simulink model "sim_yawrate"  (R2022b)
settings: Solver=VariableStepAuto  StartTime=0.0  StopTime=10.0  RelTol=1e-3
libraries: cstblocks x1
settings Model: Creator=studenti  LastModifiedBy=tonegas
settings SolverCC: AlgebraicLoopSolver=TrustRegion
settings DebuggingCC: UnconnectedInputMsg=warning  UnconnectedOutputMsg=warning  UnconnectedLineMsg=warning  SFMachineParentedDataDiag=warning
settings ModelReferenceCC: EnableRefExpFcnMdlSchedulingChecks=on

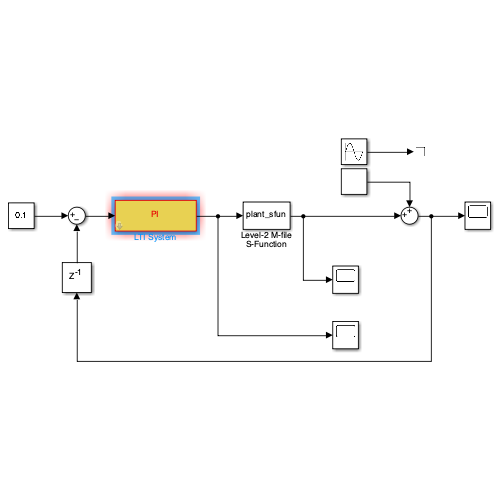
[thumbnail: Simulink's stored preview of the top-level diagram]
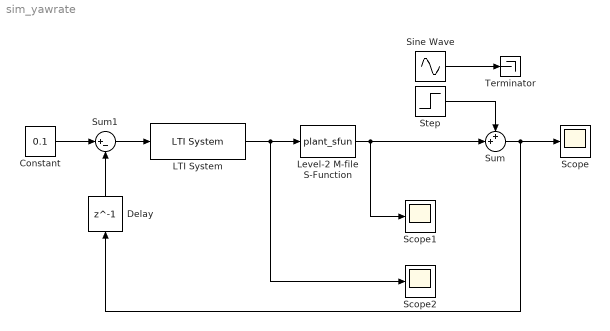
== system sim_yawrate ==
  Constant : Constant  Value=0.1
  Delay : Delay  DelayLength=1  InitialCondition=0
  LTI System : cstblocks/LTI System  sys=PI  IC=[]
  Level-2 M-file S-Function : M-S-Function  FunctionName=plant_sfun
  Scope : Scope
  Scope1 : Scope
  Scope2 : Scope
  Sine Wave : Sin  Frequency=0.5  SampleTime=0
  Step : Step  After=0.05  SampleTime=0
  Sum : Sum  Inputs=++|
  Sum1 : Sum  Inputs=|+-
  Terminator : Terminator
  wires:
  LTI System/1 -> Level-2 M-file S-Function/1, Scope2/1
  Constant/1 -> Sum1/1
  Level-2 M-file S-Function/1 -> Scope1/1, Sum/2
  Step/1 -> Sum/1
  Sum1/1 -> LTI System/1
  Sine Wave/1 -> Terminator/1
  Sum/1 -> Delay/1, Scope/1
  Delay/1 -> Sum1/2
